simulink model "Test01_SIG"  (Simulink 7.9)
settings: Solver=ode4  StartTime=0.0  StopTime=TMax  FixedStep=DT  MaxStep=DT  RelTol=1e-3
values from neighbouring files (symbols this model uses):
  GBRatio = 22.5    [Run_Test01_SIG.m]
  GenEff = 100.0    (= 100)    [Run_Test01_SIG.m]
  SIG_POTq = SIG_RtTq*SIG_PORt    (= 2735.8)    [Run_Test01_SIG.m]
  SIG_Slop = SIG_RtTq/(SIG_RtSp - SIG_SySp)    (= 719.696022001)    [Run_Test01_SIG.m]
  SIG_SySp = SIG_SySp*pi/30    (= 125.663706144)    [Run_Test01_SIG.m]
undefined symbols (not defined in the file or in its folder): OutList, strmatch
settings Model: Creator=bjonkman  LastModifiedBy=bjonkman
settings DataIOCC: LimitDataPoints=off  SaveOutput=off  SaveTime=off  SignalLoggingName=sigsOut
settings DebuggingCC: SaveWithParameterizedLinksMsg=none  SignalResolutionControl=TryResolveAllWithWarning  SolverPrmCheckMsg=none  MultiTaskDSMMsg=warning  MultiTaskCondExecSysMsg=none  FcnCallInpInsideContextMsg=Use local settings  StrictBusMsg=None
settings HardwareCC: TargetUnknown=on
settings RTWCC: IncludeERTFirstTime=on
settings GRTTargetCC: ModelReferenceCompliant=off  ParMdlRefBuildCompliant=off  CompOptLevelCompliant=off  ConcurrentExecutionCompliant=off  CombineOutputUpdateFcns=off  MatFileLogging=off  GRTInterface=on

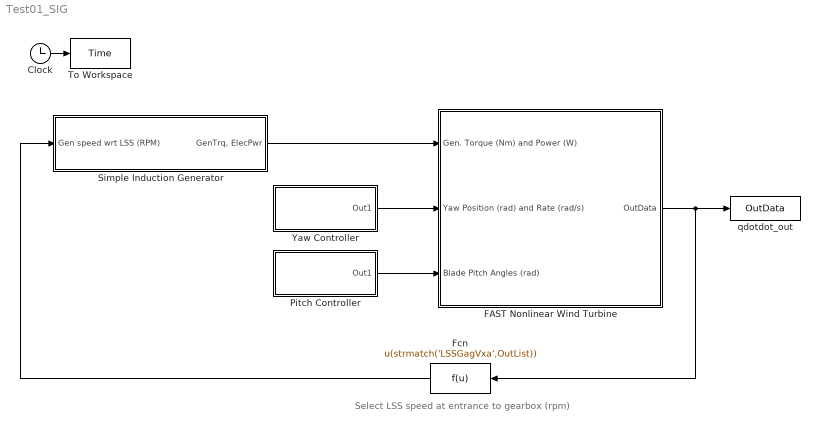
== system Test01_SIG ==
  note: Select LSS speed at entrance to gearbox (rpm)
  Clock : Clock
  FAST Nonlinear Wind Turbine : Subsystem  mask(FAST Nonlinear Wind Turbine){}
      mask help: This block contains the FAST S-Function.
      mask init:
      | clear FAST_SFunc
  Fcn : Fcn  Expr=u(strmatch('LSSGagVxa',OutList))
  Pitch Controller : Subsystem
  Simple Induction Generator : Subsystem
  To Workspace : ToWorkspace  VariableName=Time  SampleTime=-1
  Yaw Controller : Subsystem
  qdotdot_out : ToWorkspace  VariableName=OutData  SampleTime=-1
  wires:
  Clock/1 -> To Workspace/1
  FAST Nonlinear Wind Turbine/1(OutData) -> qdotdot_out/1, Fcn/1
  Simple Induction Generator/1("GenTrq, ElecPwr") -> FAST Nonlinear Wind Turbine/1(Gen. Torque (Nm) and Power (W))
  Yaw Controller/1(Out1) -> FAST Nonlinear Wind Turbine/2(Yaw Position (rad) and Rate (rad/s))
  Pitch Controller/1(Out1) -> FAST Nonlinear Wind Turbine/3(Blade Pitch Angles (rad))
  Fcn/1 -> Simple Induction Generator/1(Gen speed wrt LSS (RPM))

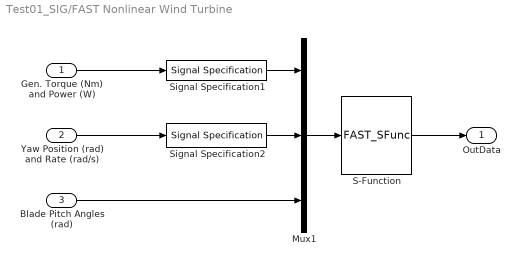
== system Test01_SIG/FAST Nonlinear Wind Turbine ==
  Gen. Torque (Nm) and Power (W) : Inport
  Yaw Position (rad) and Rate (rad/s) : Inport  Port=2
  Blade Pitch Angles (rad) : Inport  Port=3
  Mux1 : Mux  Inputs=3
  S-Function : S-Function  FunctionName=FAST_SFunc  Parameters=FAST_InputFileName, TMax, 0  EnableBusSupport=off
  Signal Specification1 : SignalSpecification  OutDataTypeStr=double  Dimensions=2
  Signal Specification2 : SignalSpecification  OutDataTypeStr=double  Dimensions=2
  OutData : Outport
  wires:
  Gen. Torque (Nm) and Power (W)/1 -> Signal Specification1/1
  S-Function/1 -> OutData/1
  Mux1/1 -> S-Function/1
  Blade Pitch Angles (rad)/1 -> Mux1/3
  Yaw Position (rad) and Rate (rad/s)/1 -> Signal Specification2/1
  Signal Specification1/1 -> Mux1/1
  Signal Specification2/1 -> Mux1/2

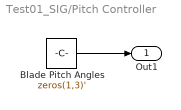
== system Test01_SIG/Pitch Controller ==
  Blade Pitch Angles : Constant  Value=zeros(1,3)'
  Out1 : Outport
  wires:
  Blade Pitch Angles/1 -> Out1/1

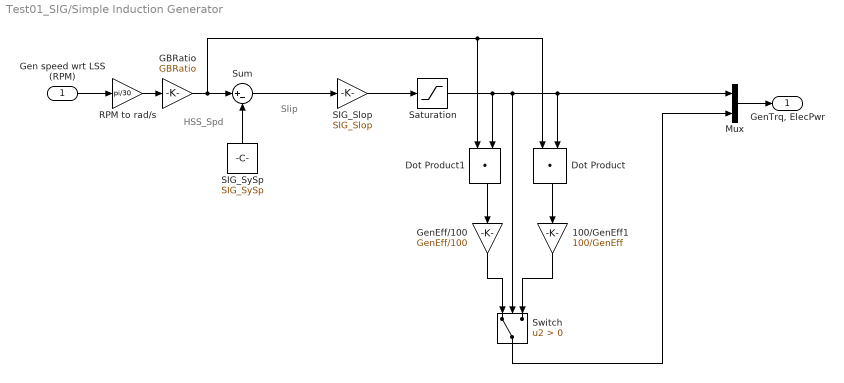
== system Test01_SIG/Simple Induction Generator ==
  note: HSS_Spd
  note: Slip
  Gen speed wrt LSS (RPM) : Inport
  100/GenEff1 : Gain  Gain=100/GenEff  SaturateOnIntegerOverflow=on  OutDataTypeStr=Inherit: Same as input  ParamDataTypeStr=Inherit: Same as input
  Dot Product : DotProduct  InputSameDT=on  OutDataTypeStr=Inherit: Inherit via internal rule
  Dot Product1 : DotProduct  InputSameDT=on  OutDataTypeStr=Inherit: Inherit via internal rule
  GBRatio : Gain  Gain=GBRatio  SaturateOnIntegerOverflow=on  OutDataTypeStr=Inherit: Same as input  ParamDataTypeStr=Inherit: Same as input
  GenEff/100 : Gain  Gain=GenEff/100  SaturateOnIntegerOverflow=on  OutDataTypeStr=Inherit: Same as input  ParamDataTypeStr=Inherit: Same as input
  Mux : Mux  Inputs=2
  RPM to rad/s : Gain  Gain=pi/30  SaturateOnIntegerOverflow=on  OutDataTypeStr=Inherit: Same as input  ParamDataTypeStr=Inherit: Same as input
  SIG_Slop : Gain  Gain=SIG_Slop  SaturateOnIntegerOverflow=on  OutDataTypeStr=Inherit: Same as input  ParamDataTypeStr=Inherit: Same as input
  SIG_SySp : Constant  Value=SIG_SySp
  Saturation : Saturate  UpperLimit=SIG_POTq  LowerLimit=-(SIG_POTq)
  Sum : Sum  Inputs=|+-  SaturateOnIntegerOverflow=on
  Switch : Switch  Criteria=u2 > Threshold  SaturateOnIntegerOverflow=on
  "GenTrq, ElecPwr" : Outport
  wires:
  SIG_SySp/1 -> Sum/2
  GBRatio/1 -> Sum/1, Dot Product/1, Dot Product1/1
  Sum/1 -> SIG_Slop/1
  SIG_Slop/1 -> Saturation/1
  Dot Product/1 -> 100/GenEff1/1
  100/GenEff1/1 -> Switch/3
  GenEff/100/1 -> Switch/1
  Dot Product1/1 -> GenEff/100/1
  Saturation/1 -> Dot Product1/2, Dot Product/2, Mux/1, Switch/2
  Mux/1 -> "GenTrq, ElecPwr"/1
  RPM to rad/s/1 -> GBRatio/1
  Switch/1 -> Mux/2
  Gen speed wrt LSS (RPM)/1 -> RPM to rad/s/1

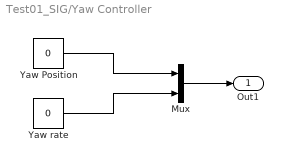
== system Test01_SIG/Yaw Controller ==
  Mux : Mux  Inputs=2
  Yaw Position : Constant  Value=0
  Yaw rate : Constant  Value=0
  Out1 : Outport
  wires:
  Mux/1 -> Out1/1
  Yaw Position/1 -> Mux/1
  Yaw rate/1 -> Mux/2
